simulink library "Wall_basic"  (R2013b)
settings: Solver=ode45  StartTime=0.0  StopTime=10.0  RelTol=1e-3
undefined symbols (not defined in the file): cond, cwall, d, dactive, rho, t0, tau
settings Model: Creator=drhf  LastModifiedBy=drhf

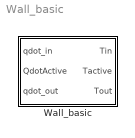
== system Wall_basic ==
  Wall_basic : Subsystem  mask(Wall basic){tau=tau, t0=t0, d=d, dactive=dactive, cond=cond, cwall=cwall, rho=rho}
      mask prompts: tau "Time constant in s"; t0 "Initial temperature in °C"; d "Thickness of layers in m"; dactive "Depth of active layer(s) in m"; cond "Conductivity of layer material in W/m/K"; cwall "Capacity of layer material in J/kg/K"; rho "Density of layer material in kg/m³"
      mask help: Basic model of a wall using a multilayer Beuken model.
      mask Help: web(fullfile(path_carnot('help'),'Wall_basic.html'),'-helpbrowser')

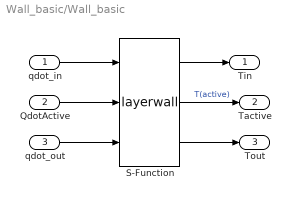
== system Wall_basic/Wall_basic ==
  qdot_in : Inport
  QdotActive : Inport  Port=2
  qdot_out : Inport  Port=3
  S-Function : S-Function  FunctionName=layerwall  Parameters=tau, t0, d, cond, cwall, rho, dactive  EnableBusSupport=off
  Tin : Outport
  Tactive : Outport  Port=2
  Tout : Outport  Port=3
  wires:
  S-Function/3 -> Tout/1
  qdot_out/1 -> S-Function/3
  S-Function/2 -> Tactive/1  "T(active)"
  QdotActive/1 -> S-Function/2
  S-Function/1 -> Tin/1
  qdot_in/1 -> S-Function/1
